simulink model "model2"  (R2025b)
settings: Solver=FixedStepAuto  StartTime=0.0  StopTime=10.0  RelTol=1e-3
values from neighbouring files (symbols this model uses):
  Thres_T = 30.0    [model2.sldd]
settings Model: DataDictionary=model2.sldd  Creator=eren  LastModifiedBy=eren
settings OptimizationCC: DefaultParameterBehavior=Inlined  UseDivisionForNetSlopeComputation=on  GainParamInheritBuiltInType=on  UseFloatMulNetSlope=on  InlineInvariantSignals=on  PassReuseOutputArgsAs=Individual arguments  ZeroExternalMemoryAtStartup=off  ZeroInternalMemoryAtStartup=off  NoFixptDivByZeroProtection=on  EfficientFloat2IntCast=on  LifeSpan=1  OptimizeBlockOrder=speed  DifferentSizesBufferReuse=on  EfficientTunableParamExpr=on
settings DebuggingCC: ParameterTunabilityLossMsg=error
settings HardwareCC: ProdBitPerPointer=32.0  ProdBitPerSizeT=32.0  ProdBitPerPtrDiffT=32.0  ProdLargestAtomicInteger=Long  ProdLargestAtomicFloat=Double  ProdWordSize=32.0  ProdLongLongMode=on  ProdHWDeviceType=ARM Compatible->ARM Cortex-M
settings SFSimCC: MATLABDynamicMemAlloc=off
settings RTWCC: SystemTargetFile=ert.tlc  TemplateMakefile=ert_default_tmf  Description=Embedded Coder
settings CodeAppCC: ForceParamTrailComments=on  IgnoreCustomStorageClasses=off  OperatorAnnotations=on  SimulinkDataObjDesc=on  SFDataObjDesc=on  CustomSymbolStrGlobalVar=rt$N$M  CustomSymbolStrType=$N$M  CustomSymbolStrFcn=$N$M$F  CustomSymbolStrMacro=$N$M  InsertBlockDesc=on
settings ERTTargetCC: ERTCustomFileTemplate=example_file_process.tlc  ERTFilePackagingFormat=CompactWithDataFile  TargetLangStandard=C99 (ISO)  GenerateSampleERTMain=on  IncludeMdlTerminateFcn=off  CombineSignalStateStructs=on  SupportAbsoluteTime=off  PurelyIntegerCode=on  SupportNonFinite=off  SupportComplex=off  SupportContinuousTime=on

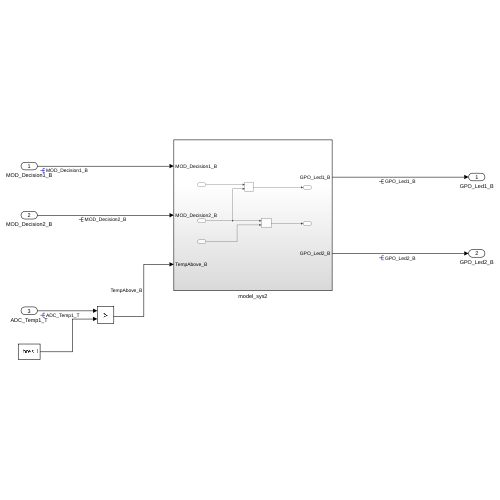
[thumbnail: Simulink's stored preview of the top-level diagram]
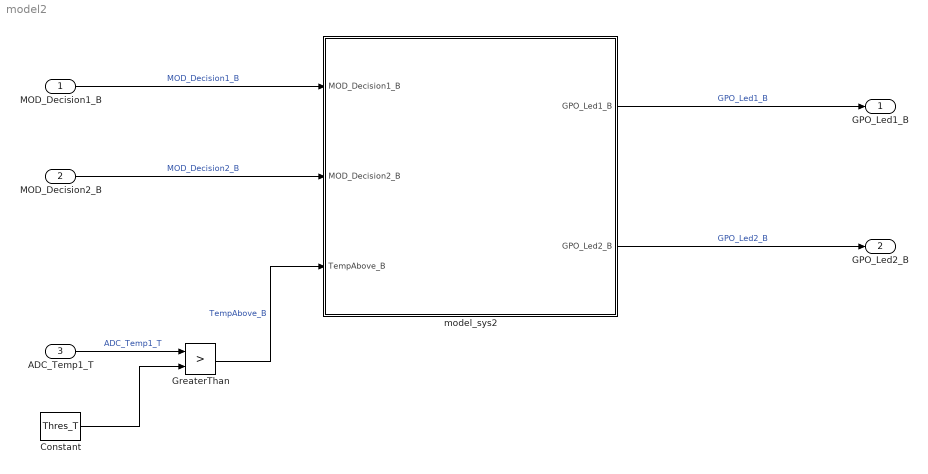
== system model2 ==
  MOD_Decision1_B : Inport
  MOD_Decision2_B : Inport  Port=2
  ADC_Temp1_T : Inport  Port=3
  Constant : Constant  Value=Thres_T
  GreaterThan : RelationalOperator  Operator=>  OutDataTypeStr=boolean  RndMeth=Simplest  InputSameDT=off
  model_sys2 : Subsystem
  GPO_Led1_B : Outport
  GPO_Led2_B : Outport  Port=2
  wires:
  MOD_Decision1_B/1 -> model_sys2/1(MOD_Decision1_B)  "MOD_Decision1_B"
  MOD_Decision2_B/1 -> model_sys2/2(MOD_Decision2_B)  "MOD_Decision2_B"
  ADC_Temp1_T/1 -> GreaterThan/1  "ADC_Temp1_T"
  Constant/1 -> GreaterThan/2
  GreaterThan/1 -> model_sys2/3(TempAbove_B)  "TempAbove_B"
  model_sys2/1(GPO_Led1_B) -> GPO_Led1_B/1  "GPO_Led1_B"
  model_sys2/2(GPO_Led2_B) -> GPO_Led2_B/1  "GPO_Led2_B"

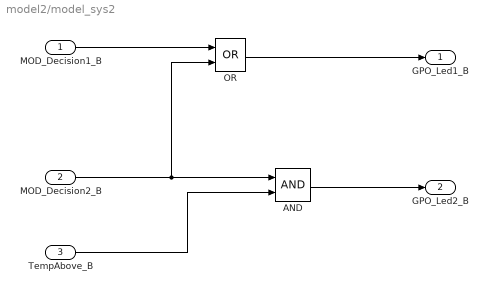
== system model2/model_sys2 ==
  MOD_Decision1_B : Inport
  MOD_Decision2_B : Inport  Port=2
  TempAbove_B : Inport  Port=3
  AND : Logic  AllPortsSameDT=off  OutDataTypeStr=boolean
  OR : Logic  Operator=OR  AllPortsSameDT=off  OutDataTypeStr=boolean
  GPO_Led1_B : Outport
  GPO_Led2_B : Outport  Port=2
  wires:
  MOD_Decision1_B/1 -> OR/1
  TempAbove_B/1 -> AND/2
  MOD_Decision2_B/1 -> OR/2, AND/1
  AND/1 -> GPO_Led2_B/1
  OR/1 -> GPO_Led1_B/1
